simulink model "model"  (R2019a)
settings: Solver=ode45  StartTime=0.0  StopTime=20  MaxStep=0.01  RelTol=1e-3  EnableMultiTasking=on
settings Model: Creator=duchn  LastModifiedBy=dn15825
settings DataIOCC: LimitDataPoints=on  SaveFormat=Array  ReturnWorkspaceOutputs=off
settings OptimizationCC: LifeSpan=inf
settings DebuggingCC: SolverPrmCheckMsg=warning  InitInArrayFormatMsg=none  SFUnexpectedBacktrackingDiag=warning  SFNoUnconditionalDefaultTransitionDiag=warning  SFExecutionAtInitializationDiag=none  ArithmeticOperatorsInVariantConditions=warning
settings HardwareCC: ProdBitPerPointer=32  ProdBitPerSizeT=32  ProdBitPerPtrDiffT=32  ProdLargestAtomicFloat=None  ProdIntDivRoundTo=Undefined  ProdEndianess=Unspecified  ProdWordSize=32  ProdHWDeviceType=32-bit Generic
settings ModelReferenceCC: PropagateSignalLabelsOutOfModel=off
settings SFSimCC: SimUseLocalCustomCode=off
settings RTWCC: RTWUseLocalCustomCode=off
settings CodeAppCC: StateflowObjectComments=on
settings GRTTargetCC: TargetLangStandard=C89/C90 (ANSI)  GeneratePreprocessorConditionals=Disable all
settings ConfigComp: CovMetricSettings=dw  CovHtmlReporting=on  CovSaveCumulativeToWorkspaceVar=on  CovSaveSingleToWorkspaceVar=on  CovExternalEMLEnable=off  CovSFcnEnable=off

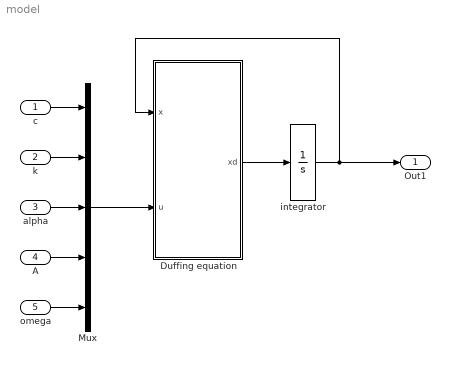
== system model ==
  c : Inport
  k : Inport  Port=2
  alpha : Inport  Port=3
  A : Inport  Port=4
  omega : Inport  Port=5
  Duffing equation : MATLAB Function  TreatAsAtomicUnit=on
  Mux : Mux  Inputs=5
  integrator : Integrator  InitialCondition=[0 0 0 1]
  Out1 : Outport
  wires:
  Duffing equation/1(xd) -> integrator/1
  integrator/1 -> Duffing equation/1(x), Out1/1
  c/1 -> Mux/1
  k/1 -> Mux/2
  alpha/1 -> Mux/3
  A/1 -> Mux/4
  omega/1 -> Mux/5
  Mux/1 -> Duffing equation/2(u)

== matlab function model/Duffing equation ==
  data: x input; u input; xd output
function xd = equations_of_motion(x,u)

x1 = x(1); % x
x2 = x(2); % x_dot
x3 = x(3); x4 = x(4); % sin and cos terms for the harmonic oscillator

% Harmonic oscillator equations
x3dot =  x3+u(5)*x4-x3*(x3^2+x4^2); % [sin(omega*t)]dot
x4dot = -u(5)*x3+x4-x4*(x3^2+x4^2); % [cos(omega*t)]dot

c=u(1); k=u(2); alpha=u(3); A=u(4); omega=u(5);

% Equation of motion - Duffing system:
% xdotdot + c*xdot + k*x + alpha*x^3  = A*cos(omega*t)
xDotDot = -c*x2-k*x1-alpha*x1^3+A*x4; 

% Output the state derivatives
xd = [x2; xDotDot; x3dot; x4dot];
